simulink model "tqdtqr_rebuild_V3"  (R2021b)
settings: Solver=VariableStepAuto  StartTime=0.0  StopTime=10.0  RelTol=1e-3
undefined symbols (not defined in the file): ATQD_AfterTqMinGain_X_Deg, ATQD_APSCreepBaseTqD_X_kph, ATQD_APSCreepBaseTqD_Y_Deg, ATQD_APSCreepBaseTqR_X_kph, ATQD_APSCreepBaseTqR_Y_Deg, ATQD_APSCreepIterm_X_kph, ATQD_APSCreepIterm_Y_kph, ATQD_APSCreepPterm_X_kph, ATQD_APSCreepPterm_Y_kph, ATQD_APSDecReq_X_kph, ATQD_APSDecReq_Y_mps2, ATQD_APSDecReqCMD_X_kph, ATQD_APSDecReqTs_X_pct, ATQD_APSDecTimeGain_X_Deg, ATQD_APSDecTimeGain_Y_s, ATQD_APSReqLowSpd_X_Deg, ATQD_AutoHoldReleaseBPS_X_Deg, ATQD_AWDLoadTrqnsGain_X_kg, ATQD_AWDLoadTrqnsGain_Y_pct, ATQD_BOSEnBPSPosn_X_kph, ATQD_BOSMap_X_rpm, ATQD_BOSMap_Y_pct, ATQD_CreepBaseTqD_X_kph, ATQD_CreepBaseTqD_Y_Deg, ATQD_CreepBaseTqR_X_kph, ATQD_CreepBaseTqR_Y_Deg, ATQD_CreepBPSDisPosn_X_Deg, ATQD_CreepBPSDisPosnR_X_Deg, ATQD_CreepBPSEnPosn_X_Deg, ATQD_CreepBPSEnPosnR_X_Deg, ATQD_CreepDeltaTq_X_kph, ATQD_CreepIterm_X_kph, ATQD_CreepIterm_Y_kph, ATQD_CreepItermMaxLimit_X_pct, ATQD_CreepPreloadTime_X_kph, ATQD_CreepPreloadTq_X_kph, ATQD_CreepPreloadTq_Y_s, ATQD_CreepProtTq_X_Deg, ATQD_CreepPterm_X_kph, ATQD_CreepPterm_Y_kph, ATQD_CreepRrTqSpRat_X_rpm, ATQD_CreepRrTqSpRat_Y_Nm, ATQD_CreepTargetSpdD_X_pct, ATQD_CreepTargetSpdR_X_pct, ATQD_CreepUpLimitTq_X_rpm, ATQD_DecIneOPDHoldEnDelay_X_Deg, ATQD_DecIneOPDHoldEnDelay_Y_bar, ATQD_ECOTqMapD_X_rpm, ATQD_ECOTqMapD_Y_pct, ATQD_EMTqMapD_X_rpm, ATQD_EMTqMapD_Y_pct, ATQD_EOPDTqMapDCon_X_rpm, ATQD_EOPDTqMapDCon_Y_Deg, ATQD_EstInitVehWeight_X_c, ATQD_FAfterTqCMDGain_X_rpm, ATQD_FAfterTqCMDGain_Y_pct, ATQD_ForceLowSpd_X_Deg, ATQD_ForcePLimitSpd_X_Deg, ATQD_FrLossMAPLowV_X_rpm, ATQD_FrLossMAPLowV_Y_Nm ... (+949)
libraries: simulink x235, hcu_lib x208, tqr x63, tqd x6
(part 7 of 37)

== system tqdtqr_rebuild_V3/Output_Convert/Signal for ESC ==
  note: Front/Rear MCU error status signals
  note: Front/Raer EDU actual torque (After Gearbox) calculation
  note: Front/Rear EDU rolling regen torque calculation
  note: Driving torque reduction permission status
  note: Front/Rear EDU speed (After Gearbox) calculation
  BSCPIn_outputs : Inport
  BInpConvert_outputs : Inport  Port=2
  BMain_outputs : Inport  Port=3
  AND1 : Logic  AllPortsSameDT=off  OutDataTypeStr=boolean
  AND2 : Logic  AllPortsSameDT=off  OutDataTypeStr=boolean
  Abs{,1..3} (4 alike) : Abs
  Bus Selector : BusSelector  OutputSignals=VINP_FrEDURealTMTq_Nm,VINP_FrntAxlTrqReqBrk_Nm,VVMC_ADASActive_flg,VINP_FrRBCActive_flg,VVMC_ACCRequiredAccel_mps2,VINP_RrEDURealTMTq_Nm,VINP_RearAxlTrqReqBrk_Nm,VINP_RrRBCActive_flg,VINP_FrTMSpd_rpm,VINP_RrTMSpd_rpm,VPMM_DrivetrainSelect_enum,VDDM_RegenErrCFS_flg,VINP_HVBattSOC_pct
  Bus Selector1 : BusSelector  OutputSignals=VTQD_GearActualPosn_enum,VTQD_RollRegenEnable_flg
  Bus Selector2 : BusSelector  OutputSignals=VTQD_AfterAvailableTqDemFr_Nm,VTQD_AfterAvailableTqDemRr_Nm,VTQD_DriverWhlTqDem_Nm,VTQR_ActualFEDUWhlTqReq_Nm,VTQR_NoABSFEDUWhlTqReq_Nm,VTQR_ActualREDUWhlTqReq_Nm,VTQR_NoABSREDUWhlTqReq_Nm
  Constant1 : Constant  Value=KTQD_AvailBRgnTqVSOC_pct
  Constant{7,10,23,25,45,47..48,50} (8 alike) : Constant  Value=ZERO_FLOAT
  Constant{3,5,8,11,34,42} (6 alike) : Constant  Value=FALSE
  Constant{2,4,9,12,29,40} (6 alike) : Constant  Value=TRUE
  Constant13 : Constant  Value=KTQD_BRegenCalEnTq_Nm
  Constant{14,16,18,20} (4 alike) : Constant  Value=eps
  Constant15 : Constant  Value=KTQD_AvailBRgnTqVSOC_pct
  Constant{17,19,21..22,24,26,44,52} (8 alike) : Constant  Value=ONE_FLOAT
  Constant27 : Constant  Value=KTQD_FrAvailBRgnTqV_flg_ovrdflg
  Constant28 : Constant  Value=KTQD_FrAvailBRgnTqV_flg_ovrdval
  Constant30 : Constant  Value=KTQD_RrAvailBRgnTqV_flg_ovrdflg
  Constant31 : Constant  Value=KTQD_RrAvailBRgnTqV_flg_ovrdval
  Constant32 : Constant  Value=KTQD_DecideEDUActTqSW_flg
  Constant33 : Constant  Value=KTQD_DecideEDUActTqSW_flg
  Constant35 : Constant  Value=ENUM_DRIVETRAIN_AWD
  Constant36 : Constant  Value=ENUM_DRIVETRAIN_FWD
  Constant37 : Constant  Value=ENUM_DRIVETRAIN_AWD
  Constant38 : Constant  Value=ENUM_DRIVETRAIN_RWD
  Constant39 : Constant  Value=KTQD_BRegenCalEnTq_Nm
  Constant41 : Constant  Value=ENUM_GEARACTUALPOSN_R
  Constant43 : Constant  Value=KVMC_ACCReqCMdBond_mps2
  Constant46 : Constant  Value=MINUSONE_FLOAT
  Constant49 : Constant  Value=KVMC_ACCReqCMdBond_mps2
  Constant51 : Constant  Value=ENUM_GEARACTUALPOSN_R
  Constant53 : Constant  Value=MINUSONE_FLOAT
  Constant6 : Constant  Value=KTQD_PTCSPermSta_flg
  Data Type Conversion{1..3,5..7} (6 alike) : DataTypeConversion  OutDataTypeStr=single
  Delay{,1..3} (4 alike) : Delay  DelayLength=1
  Divide{,1,3,5} (4 alike) : Product  Inputs=*/
  Divide{2,4,6..7} (4 alike) : Product  Inputs=**
  Equal{,1..3,8..9} (6 alike) : RelationalOperator  Operator=<  OutDataTypeStr=boolean  RndMeth=Simplest
  Equal{4..7,10..11} (6 alike) : RelationalOperator  Operator===  OutDataTypeStr=boolean  RndMeth=Simplest
  Gain1 : Gain  Gain=1/KTQD_FrTMTotalGearRatio_gain
  Gain{4,6..7,10} (4 alike) : Gain  Gain=KTQD_RrTMTotalGearRatio_gain
  Gain2 : Gain  Gain=1/KTQD_RrTMTotalGearRatio_gain
  Gain{3,5,8..9} (4 alike) : Gain  Gain=KTQD_FrTMTotalGearRatio_gain
  Logical Operator : Logic  Operator=OR  AllPortsSameDT=off  OutDataTypeStr=boolean
  Logical Operator1 : Logic  AllPortsSameDT=off  OutDataTypeStr=boolean
  Logical Operator2 : Logic  AllPortsSameDT=off  OutDataTypeStr=boolean
  Max : MinMax  Function=max  Inputs=2
  Max1 : MinMax  Function=max  Inputs=2
  OR{,1..7} (8 alike) : Logic  Operator=OR  AllPortsSameDT=off  OutDataTypeStr=boolean
  Product : Product
  Product1 : Product
  Relational Operator{,1,4..5} (4 alike) : RelationalOperator  Operator=<=  OutDataTypeStr=boolean  RndMeth=Simplest
  Relational Operator2 : RelationalOperator  Operator=<  OutDataTypeStr=boolean  RndMeth=Simplest
  Relational Operator3 : RelationalOperator  Operator=<  OutDataTypeStr=boolean  RndMeth=Simplest
  Relational Operator6 : RelationalOperator  OutDataTypeStr=boolean  RndMeth=Simplest
  Relational Operator7 : RelationalOperator  OutDataTypeStr=boolean  RndMeth=Simplest
  Saturation : Saturate  UpperLimit=KTQD_FrBRgnCalUpLim_Nm  LowerLimit=KTQD_FrBRgnCalLowLim_Nm
      settings: AttributesFormatString=|
      | UpperLimit: %<UpperLimit>
      | LowerLimit: %<LowerLimit>
  Saturation1 : Saturate  UpperLimit=KTQD_RrBRgnCalUpLim_Nm  LowerLimit=KTQD_RrBRgnCalLowLim_Nm
      settings: AttributesFormatString=|
      | UpperLimit: %<UpperLimit>
      | LowerLimit: %<LowerLimit>
  Saturation2 : Saturate  UpperLimit=KTQD_RrEDURollRgnUpTq_Nm  LowerLimit=KTQD_RrEDURollRgnLowTq_Nm
      settings: AttributesFormatString=|
      | UpperLimit: %<UpperLimit>
      | LowerLimit: %<LowerLimit>
  Saturation3 : Saturate  UpperLimit=KTQD_FrEDURollRgnUpTq_Nm  LowerLimit=KTQD_FrEDURollRgnLowTq_Nm
  Saturation{4..7} (4 alike) : Saturate  UpperLimit=KTQD_TMTqDeviationUp_c  LowerLimit=KTQD_TMTqDeviationLow_c
      Saturation4 settings: AttributesFormatString=|
      | UpperLimit: %<UpperLimit>
      | LowerLimit: %<LowerLimit>
      Saturation5 settings: AttributesFormatString=|
      | UpperLimit: %<UpperLimit>
      | LowerLimit: %<LowerLimit>
      Saturation6 settings: LockScale=on
      Saturation6 settings: AttributesFormatString=|
      | UpperLimit: %<UpperLimit>
      | LowerLimit: %<LowerLimit>
      Saturation7 settings: AttributesFormatString=|
      | UpperLimit: %<UpperLimit>
      | LowerLimit: %<LowerLimit>
  Switch{,1..18,20..21,23} (22 alike) : Switch  Criteria=u2 ~= 0
  Switch{19,22,24..27} (6 alike) : Switch  Criteria=u2 > Threshold
  VTQD_FrEDUActTq_Nm : Outport
  VTQD_RrEDUActTq_Nm : Outport  Port=2
  VTQD_FrEDURolRgnTq_Nm : Outport  Port=3
  VTQD_RrEDURolRgnTq_Nm : Outport  Port=4
  VTQD_FrEDUSpd_rpm : Outport  Port=5
  VTQD_RrEDUSpd_rpm : Outport  Port=6
  VTQD_FrEDUSpdValid_flg : Outport  Port=7
  VTQD_FrEDUActTqValid_flg : Outport  Port=8
  VTQD_FrEDURolRgnTqValid_flg : Outport  Port=9
  VTQD_FrEDUAvailBrkRgnTqV_flg : Outport  Port=10
  VTQD_RrEDUSpdValid_flg : Outport  Port=11
  VTQD_RrEDUActTqValid_flg : Outport  Port=12
  VTQD_RrEDURolRgnTqValid_flg : Outport  Port=13
  VTQD_RrEDUAvailBrkRgnTqV_flg : Outport  Port=14
  VTQD_RgnAbnorSta_flg : Outport  Port=15
  VTQD_PTCSPermSta_flg : Outport  Port=16
  wires:
  Logical Operator/1 -> VTQD_RgnAbnorSta_flg/1  "VTQD_RgnAbnorSta_flg"
  [VINP_RrEDURealTMTq_Nm] -> Gain6/1
  Relational Operator/1 -> Switch5/2
  Saturation6/1 -> Divide6/2  "VTQD_FrARgnTqDeviation_c"
  Constant10/1 -> Relational Operator1/2
  Constant12/1 -> Switch9/1
  OR1/1 -> Switch6/2
  [VINP_FrTMSpd_rpm] -> Gain1/1
  Divide6/1 -> Switch4/1  "VTQD_FrARegenCal_Nm"
  Constant7/1 -> Relational Operator/2
  [VTQR_NoABSFEDUWhlTqReq_Nm] -> Divide6/1
  [VINP_FrEDURealTMTq_Nm] -> Gain5/1
  [VINP_FrEDURealTMTq_Nm] -> Gain8/1
  Relational Operator3/1 -> Switch15/2
  Constant17/1 -> Switch8/1
  Gain8/1 -> Saturation/1
  [VTQR_ActualFEDUWhlTqReq_Nm] -> Delay2/1
  Switch4/1 -> Saturation3/1
  Divide4/1 -> Data Type Conversion7/1  "VTQD_RrBRegenCal_Nm"
  Saturation4/1 -> Divide2/2
  Constant22/1 -> Switch13/1
  Relational Operator2/1 -> Switch14/2
  Divide2/1 -> Data Type Conversion1/1  "VTQD_FrBRegenCal_Nm"
  OR/1 -> Switch4/2
  [VTQD_DriverWhlTqDem_Nm] -> Relational Operator1/1
  Data Type Conversion5/1 -> VTQD_FrEDUSpd_rpm/1  "VTQD_FrEDUSpd_rpm"
  Constant23/1 -> Relational Operator2/2
  [VTQR_ActualFEDUWhlTqReq_Nm] -> Delay/1
  Gain3/1 -> Divide/1
  Switch12/1 -> Switch14/3, Relational Operator2/1  "VTQD_FrTMTqDeviation_c"
  Data Type Conversion6/1 -> VTQD_RrEDUSpd_rpm/1  "VTQD_RrEDUSpd_rpm"
  Switch15/1 -> Saturation5/1  "VTQD_ActRrTMTqDeviation_c"
  Gain6/1 -> Divide5/1
  [VINP_RrEDURealTMTq_Nm] -> Gain7/1
  Data Type Conversion3/1 -> VTQD_RrEDURolRgnTq_Nm/1  "VTQD_RrEDURolRgnTq_Nm"
  Data Type Conversion2/1 -> VTQD_FrEDURolRgnTq_Nm/1  "VTQD_FrEDURolRgnTq_Nm"
  Constant49/1 -> Equal9/2
  Constant9/1 -> Switch5/1
  Max1/1 -> Divide4/1
  [VVMC_ADASActive_flg] -> Switch18/2
  Relational Operator6/1 -> OR6/1
  Equal1/1 -> Switch8/2
  [VVMC_ADASActive_flg] -> Switch19/2
  Equal11/1 -> Switch27/2
  Equal5/1 -> OR2/2
  Equal7/1 -> OR3/2
  [VPMM_DrivetrainSelect_enum] -> Equal4/1
  Divide1/1 -> Saturation6/1
  Abs2/1 -> Equal/1
  Equal6/1 -> OR3/1
  Constant35/1 -> Equal4/2
  Logical Operator1/1 -> Switch3/2
  [VINP_FrntAxlTrqReqBrk_Nm] -> Max/2
  Constant26/1 -> Switch15/1
  Switch3/1 -> Logical Operator/1, VTQD_FrEDURolRgnTqValid_flg/1, VTQD_FrEDUActTqValid_flg/1, VTQD_FrEDUSpdValid_flg/1
  [VINP_HVBattSOC_pct] -> Relational Operator7/1
  Switch9/1 -> OR1/2  "VTQD_RrWhlTqDemNeg_flg"
  Switch26/1 -> Product/1
  [VINP_FrEDURealTMTq_Nm] -> Gain9/1
  Gain5/1 -> Divide1/1
  Switch10/1 -> Product1/2
  [VVMC_ADASActive_flg] -> Switch22/2
  [VTQD_DriverWhlTqDem_Nm] -> Relational Operator/1
  Constant2/1 -> Switch2/1
  [VTQR_NoABSREDUWhlTqReq_Nm] -> Switch25/3
  [VINP_FrEDURealTMTq_Nm] -> Gain3/1
  Switch16/1 -> VTQD_FrEDUAvailBrkRgnTqV_flg/1  "VTQD_FrEDUAvailBrkRgnTqV_flg"
  OR2/1 -> Logical Operator1/1
  [VINP_RrEDURealTMTq_Nm] -> Gain10/1
  [VINP_RrEDURealTMTq_Nm] -> Gain4/1
  Gain7/1 -> Saturation1/1
  [VINP_RearAxlTrqReqBrk_Nm] -> Max1/2
  Product1/1 -> VTQD_RrEDUActTq_Nm/1  "VTQD_RrEDUActTq_Nm"
  [VTQD_GearActualPosn_enum] -> Equal11/1
  [VTQD_AfterAvailableTqDemFr_Nm] -> Switch24/1
  Constant29/1 -> Switch20/3
  [VVMC_ADASActive_flg] -> Switch1/2
  Gain10/1 -> Max1/1
  Constant25/1 -> Relational Operator3/2
  Constant32/1 -> Switch24/2
  Constant15/1 -> Relational Operator7/2
  Constant51/1 -> Equal11/2
  Divide3/1 -> Switch13/3
  Switch27/1 -> Product1/1
  Constant53/1 -> Switch27/1
  Switch18/1 -> Switch10/1
  [VTQD_GearActualPosn_enum] -> Equal10/1
  Relational Operator5/1 -> OR4/2
  Switch8/1 -> Divide1/2
  Constant18/1 -> Equal1/2
  [VTQD_RollRegenEnable_flg] -> OR1/1
  [VVMC_ADASActive_flg] -> OR4/1
  Saturation1/1 -> Switch23/3
  Equal/1 -> Switch12/2
  Constant33/1 -> Switch25/2
  [VTQD_RollRegenEnable_flg] -> OR/1
  Constant6/1 -> VTQD_PTCSPermSta_flg/1  "VTQD_PTCSPermSta_flg"
  Constant24/1 -> Switch14/1
  Constant44/1 -> Switch26/3
  Switch25/1 -> Relational Operator5/1
  Delay3/1 -> Abs1/1, Switch11/3
  Data Type Conversion1/1 -> Switch1/3
  [VTQR_NoABSFEDUWhlTqReq_Nm] -> Switch24/3
  OR7/1 -> Switch20/2
  Switch2/1 -> VTQD_RrEDUActTqValid_flg/1, Logical Operator/2, VTQD_RrEDUSpdValid_flg/1, VTQD_RrEDURolRgnTqValid_flg/1
  [VPMM_DrivetrainSelect_enum] -> Equal6/1
  Product/1 -> VTQD_FrEDUActTq_Nm/1  "VTQD_FrEDUActTq_Nm"
  Constant40/1 -> Switch21/3
  Saturation2/1 -> Data Type Conversion3/1
  [VVMC_ADASActive_flg] -> OR5/1
  Constant5/1 -> Switch3/3
  [VVMC_ADASActive_flg] -> OR7/2
  [VTQD_AfterAvailableTqDemRr_Nm] -> Switch25/1
  Abs3/1 -> Equal2/1
  OR6/1 -> Switch21/2
  Constant31/1 -> Switch17/1
  Switch23/1 -> Switch10/3
  Switch24/1 -> Relational Operator4/1
  Gain1/1 -> Data Type Conversion5/1
  Relational Operator4/1 -> OR5/2
  [VINP_HVBattSOC_pct] -> Relational Operator6/1
  Switch7/1 -> Product/2
  Saturation5/1 -> Divide4/2
  Constant39/1 -> Relational Operator5/2
  [VVMC_ADASActive_flg] -> OR6/2
  Constant20/1 -> Equal3/2
  Switch21/1 -> Switch17/3
  [VINP_RrRBCActive_flg] -> AND1/1
  Constant1/1 -> Relational Operator6/2
  Relational Operator7/1 -> OR7/1
  Constant8/1 -> Switch5/3
  OR5/1 -> AND2/2
  Delay/1 -> Divide/2, Abs2/1
  Abs/1 -> Equal1/1
  Switch/1 -> Switch7/3
  [VVMC_ACCRequiredAccel_mps2] -> Equal9/1
  Constant48/1 -> Switch/1
  [VTQR_NoABSFEDUWhlTqReq_Nm] -> Switch19/3
  Constant16/1 -> Equal2/2
  Equal9/1 -> Switch23/2
  Constant21/1 -> Switch12/1
  Constant19/1 -> Switch11/1
  Delay1/1 -> Abs3/1, Divide3/2
  Constant14/1 -> Equal/2
  Constant46/1 -> Switch26/1
  [VINP_RrTMSpd_rpm] -> Gain2/1
  Constant50/1 -> Switch23/1
  Switch22/1 -> Switch6/3
  Saturation/1 -> Switch/3
  Logical Operator2/1 -> Switch2/2
  Constant3/1 -> Switch2/3
  Constant45/1 -> Switch22/1
  [VTQR_NoABSREDUWhlTqReq_Nm] -> Switch22/3
  Switch19/1 -> Switch4/3
  Switch1/1 -> Switch7/1
  Constant42/1 -> Switch21/1
  [VINP_FrRBCActive_flg] -> AND2/1
  [VVMC_ACCRequiredAccel_mps2] -> Equal8/1
  OR4/1 -> AND1/2
  Switch20/1 -> Switch16/3
  Switch6/1 -> Saturation2/1
  [VDDM_RegenErrCFS_flg] -> Logical Operator2/2
  AND1/1 -> Switch10/2
  AND2/1 -> Switch7/2
  Switch13/1 -> Switch15/3, Relational Operator3/1  "VTQD_RrTMTqDeviation_c"
  Constant30/1 -> Switch17/2
  Constant4/1 -> Switch3/1
  Data Type Conversion7/1 -> Switch18/3
  Switch14/1 -> Saturation4/1  "VTQD_ActFrTMTqDeviation_c"
  Switch17/1 -> VTQD_RrEDUAvailBrkRgnTqV_flg/1  "VTQD_RrEDUAvailBrkRgnTqV_flg"
  Delay2/1 -> Abs/1, Switch8/3
  Saturation3/1 -> Data Type Conversion2/1
  [VTQR_ActualREDUWhlTqReq_Nm] -> Delay3/1
  Equal10/1 -> Switch26/2
  Constant28/1 -> Switch16/1
  Divide7/1 -> Switch6/1  "VTQD_RrARegenCal_Nm"
  [VTQR_NoABSREDUWhlTqReq_Nm] -> Divide7/1
  Divide5/1 -> Saturation7/1
  Constant11/1 -> Switch9/3
  Saturation7/1 -> Divide7/2  "VTQD_RrARgnTqDeviation_c"
  Switch5/1 -> OR/2  "VTQD_FrWhlTqDemNeg_flg"
  [VPMM_DrivetrainSelect_enum] -> Equal7/1
  OR3/1 -> Logical Operator2/1
  Constant13/1 -> Relational Operator4/2
  Equal4/1 -> OR2/1
  [VINP_FrntAxlTrqReqBrk_Nm] -> Switch1/1
  Equal2/1 -> Switch13/2
  Constant52/1 -> Switch27/3
  Max/1 -> Divide2/1
  Constant38/1 -> Equal7/2
  [VINP_RearAxlTrqReqBrk_Nm] -> Switch18/1
  Constant41/1 -> Equal10/2
  Constant37/1 -> Equal6/2
  [VTQR_ActualREDUWhlTqReq_Nm] -> Delay1/1
  Constant43/1 -> Equal8/2
  Gain9/1 -> Max/1
  Relational Operator1/1 -> Switch9/2
  Switch11/1 -> Divide5/2
  Gain4/1 -> Divide3/1
  Constant27/1 -> Switch16/2
  Gain2/1 -> Data Type Conversion6/1
  Constant47/1 -> Switch19/1
  [VPMM_DrivetrainSelect_enum] -> Equal5/1
  [VDDM_RegenErrCFS_flg] -> Logical Operator1/2
  Constant34/1 -> Switch20/1
  Equal8/1 -> Switch/2
  Constant36/1 -> Equal5/2
  Abs1/1 -> Equal3/1
  Equal3/1 -> Switch11/2
  Divide/1 -> Switch12/3
  BSCPIn_outputs/1 -> Bus Selector/1
  BInpConvert_outputs/1 -> Bus Selector1/1
  BMain_outputs/1 -> Bus Selector2/1
  Bus Selector/1 -> [VINP_FrEDURealTMTq_Nm]  "<VINP_FrEDURealTMTq_Nm>"
  Bus Selector/2 -> [VINP_FrntAxlTrqReqBrk_Nm]  "<VINP_FrntAxlTrqReqBrk_Nm>"
  Bus Selector/3 -> [VVMC_ADASActive_flg]  "<VVMC_ADASActive_flg>"
  Bus Selector/4 -> [VINP_FrRBCActive_flg]  "<VINP_FrRBCActive_flg>"
  Bus Selector2/1 -> [VTQD_AfterAvailableTqDemFr_Nm]  "<VTQD_AfterAvailableTqDemFr_Nm>"
  Bus Selector/5 -> [VVMC_ACCRequiredAccel_mps2]  "<VVMC_ACCRequiredAccel_mps2>"
  Bus Selector1/1 -> [VTQD_GearActualPosn_enum]  "<VTQD_GearActualPosn_enum>"
  Bus Selector/6 -> [VINP_RrEDURealTMTq_Nm]  "<VINP_RrEDURealTMTq_Nm>"
  Bus Selector/7 -> [VINP_RearAxlTrqReqBrk_Nm]  "<VINP_RearAxlTrqReqBrk_Nm>"
  Bus Selector/8 -> [VINP_RrRBCActive_flg]  "<VINP_RrRBCActive_flg>"
  Bus Selector2/2 -> [VTQD_AfterAvailableTqDemRr_Nm]  "<VTQD_AfterAvailableTqDemRr_Nm>"
  Bus Selector/9 -> [VINP_FrTMSpd_rpm]  "<VINP_FrTMSpd_rpm>"
  Bus Selector/10 -> [VINP_RrTMSpd_rpm]  "<VINP_RrTMSpd_rpm>"
  Bus Selector/11 -> [VPMM_DrivetrainSelect_enum]  "<VPMM_DrivetrainSelect_enum>"
  Bus Selector/12 -> [VDDM_RegenErrCFS_flg]  "<VDDM_RegenErrCFS_flg>"
  Bus Selector2/3 -> [VTQD_DriverWhlTqDem_Nm]  "<VTQD_DriverWhlTqDem_Nm>"
  Bus Selector1/2 -> [VTQD_RollRegenEnable_flg]  "<VTQD_RollRegenEnable_flg>"
  Bus Selector/13 -> [VINP_HVBattSOC_pct]  "<VINP_HVBattSOC_pct>"
  Bus Selector2/4 -> [VTQR_ActualFEDUWhlTqReq_Nm]  "<VTQR_ActualFEDUWhlTqReq_Nm>"
  Bus Selector2/5 -> [VTQR_NoABSFEDUWhlTqReq_Nm]  "<VTQR_NoABSFEDUWhlTqReq_Nm>"
  Bus Selector2/6 -> [VTQR_ActualREDUWhlTqReq_Nm]  "<VTQR_ActualREDUWhlTqReq_Nm>"
  Bus Selector2/7 -> [VTQR_NoABSREDUWhlTqReq_Nm]  "<VTQR_NoABSREDUWhlTqReq_Nm>"

== system tqdtqr_rebuild_V3/Output_Convert/Signals for BCM ==
  BSCPIn_outputs : Inport
  VTQD_ARegenActive_flg : Inport  Port=2
  Bus Selector : BusSelector  OutputSignals=VINP_LongAccel_Gps
  Constant : Constant  Value=KVMC_GravityValue_mps2
  Logical Operator : Logic  AllPortsSameDT=off  OutDataTypeStr=boolean
  Product : Product
  Relay1 : Relay  OnSwitchValue=KTQD_RegBrkLPOff_c  OffSwitchValue=KTQD_RegBrkLPOn_c  OnOutputValue=0  OffOutputValue=1
      settings: AttributesFormatString=|
      | ON: %<OnSwitchValue>
      | OFF: %<OffSwitchValue>
  VTQD_ReBrakeLPReq_flg : Outport
  wires:
  BSCPIn_outputs/1 -> Bus Selector/1
  Product/1 -> Relay1/1
  [VINP_LongAccel_Gps] -> Product/2
  [VTQD_ARegenActive_flg] -> Logical Operator/1
  Constant/1 -> Product/1
  Relay1/1 -> Logical Operator/2
  Logical Operator/1 -> VTQD_ReBrakeLPReq_flg/1  "VTQD_ReBrakeLPReq_flg"
  Bus Selector/1 -> [VINP_LongAccel_Gps]  "<VINP_LongAccel_Gps>"
  VTQD_ARegenActive_flg/1 -> [VTQD_ARegenActive_flg]

== system tqdtqr_rebuild_V3/Output_Convert/Signals for MCU ==
  Constant : Constant  Value=KTQD_FrIdcMin_A
  Constant1 : Constant  Value=KTQD_FrIdcMax_A
  Constant2 : Constant  Value=KTQD_FrUdcMax_V
  Constant3 : Constant  Value=KTQD_FrUdcMin_V
  Constant4 : Constant  Value=KTQD_RrIdcMin_A
  Constant5 : Constant  Value=KTQD_RrIdcMax_A
  Constant6 : Constant  Value=KTQD_RrUdcMax_V
  Constant7 : Constant  Value=KTQD_RrUdcMin_V
  VTQD_FrIdcMin_A : Outport
  VTQD_FrIdcMax_A : Outport  Port=2
  VTQD_FrUdcMin_V : Outport  Port=3
  VTQD_FrUdcMax_V : Outport  Port=4
  VTQD_RrIdcMin_A : Outport  Port=5
  VTQD_RrIdcMax_A : Outport  Port=6
  VTQD_RrUdcMin_V : Outport  Port=7
  VTQD_RrUdcMax_V : Outport  Port=8
  wires:
  Constant6/1 -> VTQD_RrUdcMax_V/1  "VTQD_RrUdcMax_V"
  Constant2/1 -> VTQD_FrUdcMax_V/1  "VTQD_FrUdcMax_V"
  Constant/1 -> VTQD_FrIdcMin_A/1  "VTQD_FrIdcMin_A"
  Constant7/1 -> VTQD_RrUdcMin_V/1  "VTQD_RrUdcMin_V"
  Constant1/1 -> VTQD_FrIdcMax_A/1  "VTQD_FrIdcMax_A"
  Constant5/1 -> VTQD_RrIdcMax_A/1  "VTQD_RrIdcMax_A"
  Constant4/1 -> VTQD_RrIdcMin_A/1  "VTQD_RrIdcMin_A"
  Constant3/1 -> VTQD_FrUdcMin_V/1  "VTQD_FrUdcMin_V"
